simulink model "quado"  (Simulink 8.7)
settings: Solver=VariableStepAuto  SolverMode=SingleTasking  StartTime=0.0  StopTime=0.3  MaxStep=1e-4  RelTol=1e-3
libraries: powerlib x11
settings Model: Creator=BTSS  LastModifiedBy=BTSS
settings DataIOCC: LimitDataPoints=off  SaveFormat=Dataset  ReturnWorkspaceOutputs=on
settings DebuggingCC: UnderspecifiedInitializationDetection=Simplified  MergeDetectMultiDrivingBlocksExec=error  UnconnectedInputMsg=none  UnconnectedOutputMsg=none  UnconnectedLineMsg=none  SFUnexpectedBacktrackingDiag=error  SFNoUnconditionalDefaultTransitionDiag=error
settings HardwareCC: ProdBitPerPointer=64  ProdLargestAtomicFloat=Float  ProdIntDivRoundTo=Zero  ProdEndianess=LittleEndian  ProdWordSize=64  ProdHWDeviceType=Intel->x86-64 (Windows64)
settings ModelReferenceCC: EnableRefExpFcnMdlSchedulingChecks=off  PropagateSignalLabelsOutOfModel=on
settings SFSimCC: SimUseLocalCustomCode=on
settings RTWCC: RTWUseLocalCustomCode=on
settings GRTTargetCC: TargetLangStandard=C99 (ISO)
settings ConfigComp: CovMetricSettings=dwe  CovSaveCumulativeToWorkspaceVar=off  CovSaveSingleToWorkspaceVar=off  CovModelRefEnable=off  CovExternalEMLEnable=on

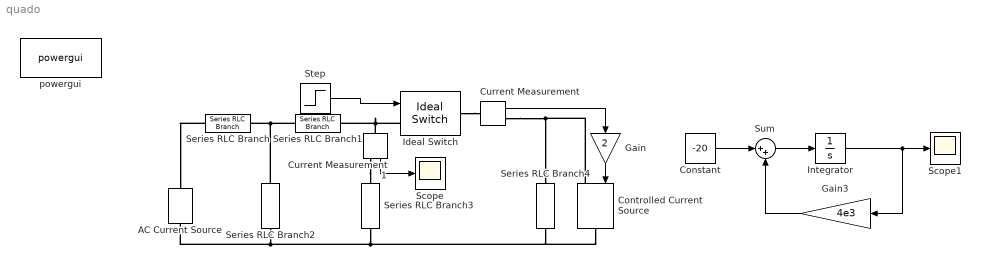
== system quado ==
  AC Current Source : powerlib/Electrical Sources/AC Current Source  Amplitude=10e-3  Phase=90  Frequency=0  SampleTime=0  Measurements=None
  Constant : Constant  Value=-20
  Controlled Current Source : powerlib/Electrical Sources/Controlled Current Source  Initialize=off  Source_Type=AC  Amplitude=0  Phase=0  Frequency=0  Measurements=None
  Current Measurement : powerlib/Measurements/Current Measurement  PhasorSimulation=off  OutputType=Complex  PSBequivalent=0
  Current Measurement1 : powerlib/Measurements/Current Measurement  PhasorSimulation=off  OutputType=Complex  PSBequivalent=0
  Gain : Gain  Gain=2
  Gain3 : Gain  Gain=4e3
  Ideal Switch : powerlib/Power Electronics/Ideal Switch  Ron=1e-9  Lon=0  IC=0  Rs=inf  Cs=inf  Measurements=off
  Integrator : Integrator  InitialCondition=5e-3
  Scope : Scope
  Scope1 : Scope
  Series RLC Branch{,1..2,4} (4 alike) : powerlib/Elements/Series RLC Branch  LConnTagsString=__new0  RConnTagsString=__new0  BranchType=R  Resistance=2e3  Inductance=1e-3  SetiL0=off  InitialCurrent=0  Capacitance=1e-6  Setx0=off  InitialVoltage=0  Measurements=None
  Series RLC Branch3 : powerlib/Elements/Series RLC Branch  LConnTagsString=__new0  RConnTagsString=__new0  BranchType=L  Resistance=2e3  Inductance=2e-3  SetiL0=off  InitialCurrent=0  Capacitance=1e-6  Setx0=off  InitialVoltage=0  Measurements=None
  Step : Step  Time=0.1  SampleTime=0
  Sum : Sum  Inputs=|++
  powergui : powerlib/powergui  Priority=1  SimulationMode=Continuous  SampleTime=50e-6  frequency=60  Iterations=50  frequencyindice=0  Pbase=100e6  ErrMax=1e-4  UnitsV=kV  UnitsW=MW  buscounter=0  FunctionMessages=off  echomessages=off  EnableUseOfTLC=off  CurrentSourceSwitches=off  DisableSnubberDevices=off  DisableRonSwitches=off  DisableVfSwitches=off  DisplayEquations=off  AutomaticDiscreteSolvers=off  SolverType=Tustin/Backward Euler (TBE)  Interpol=off  ExternalGateDelay=off  methode=off  Ts=100  x0status=blocks  SPID=on  SwTol=0  HookPort=off  NonlinearTolerance=1e-4  nMaxIteration=100  ContinueOnMaxIteration=off  RestoreLinks=warning  ResistiveCurrentMeasurement=off  Frange=[0:2:500]  Ylog=off  Xlog=on  ShowGrid=off  save=off  variable=ZData  structure=0  ZoomFFT=off  StartTime=0.0  cycles=1  DisplayStyle=1  fundamental=60  FreqAxis=off  MaxFrequency=1000  frequencyindicesteady=1  RmsSteady=1  display=off
  wires:
  Current Measurement/1 -> Gain/1
  Gain/1 -> Controlled Current Source/1
  Step/1 -> Ideal Switch/1
  Current Measurement1/1 -> Scope/1
  Constant/1 -> Sum/1
  Gain3/1 -> Sum/2
  Sum/1 -> Integrator/1
  Integrator/1 -> Scope1/1, Gain3/1
  connections:
  Series RLC Branch/LConn1 -- AC Current Source/RConn1
  Series RLC Branch1/LConn1 -- Series RLC Branch2/LConn1 -- Series RLC Branch/RConn1
  Ideal Switch/LConn1 -- Current Measurement1/LConn1 -- Series RLC Branch1/RConn1
  Series RLC Branch3/RConn1 -- Series RLC Branch4/RConn1 -- Controlled Current Source/RConn1 -- Series RLC Branch2/RConn1 -- AC Current Source/LConn1
  Current Measurement/RConn1 -- Series RLC Branch4/LConn1 -- Controlled Current Source/LConn1
  Ideal Switch/RConn1 -- Current Measurement/LConn1
  Current Measurement1/RConn1 -- Series RLC Branch3/LConn1
